simulink model "ctrlSys_mpc"  (R2025b)
settings: Solver=ode14x  StartTime=0.0  StopTime=70  FixedStep=Ts_local  RelTol=1e-4
model workspace (MAT data in the model file):
  CtrlChoice = "MPC"
values from neighbouring files (symbols this model uses):
  Ts_ctrl = 0.1    [ctrlSys.sldd]
libraries: slpidlib x1
settings Model: DataDictionary=ctrlSys.sldd  SimulationMode=accelerator  Creator=LYG  LastModifiedBy=mercer
settings SolverCC: ZeroCrossControl=DisableAll

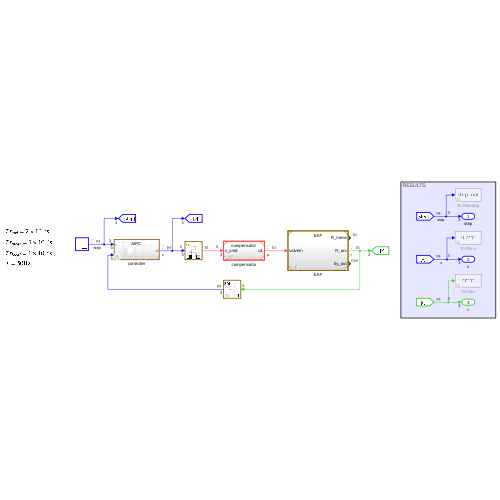
[thumbnail: Simulink's stored preview of the top-level diagram]
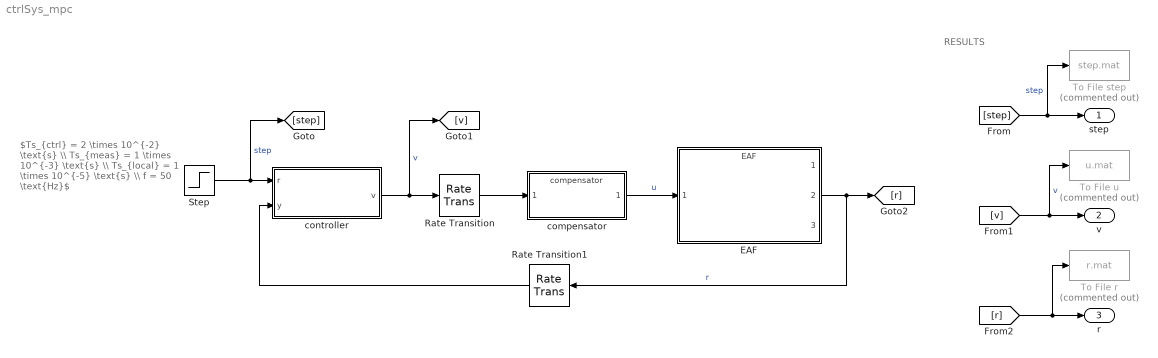
== system ctrlSys_mpc ==
  note: RESULTS
  note: $Ts_{ctrl} = 2 \times 10^{-2} \text{s} \\ Ts_{meas} = 1 \times 10^{-3} \text{s} \\ Ts_{local} = 1 \times 10^{-5} \text{s} \\ f = 50 \text{Hz}$
  EAF : ModelReference  ModelNameDialog=EAF.slx  SimulationMode=Normal  ModelReferenceVersion=1.78
  Rate Transition : RateTransition  OutPortSampleTime=Ts_local
  Rate Transition1 : RateTransition  OutPortSampleTime=Ts_ctrl
  Step : Step  Time=[35 20 50]  Before=[0.06 0.055 0.09]  After=[0.05 0.065 0.10]  SampleTime=Ts_ctrl
  To File r : ToFile  Commented=on  Filename=r.mat  MatrixName=r  SaveFormat=Timeseries
  To File step : ToFile  Commented=on  Filename=step.mat  MatrixName=step  SaveFormat=Timeseries
  To File u : ToFile  Commented=on  Filename=u.mat  MatrixName=u  SaveFormat=Timeseries
  compensator : ModelReference  ModelNameDialog=compensator.slx  SimulationMode=Normal  ModelReferenceVersion=1.22
  controller : Subsystem  Variant=on
  step : Outport
  v : Outport  Port=2
  r : Outport  Port=3
  wires:
  controller/1(v) -> [v], Rate Transition/1  "v"
  Step/1 -> controller/1(r), [step]  "step"
  Rate Transition1/1 -> controller/2(y)
  [step] -> To File step/1, step/1  "step"
  [v] -> To File u/1, v/1  "v"
  [r] -> To File r/1, r/1
  EAF/2 -> Rate Transition1/1, [r]  "r"
  Rate Transition/1 -> compensator/1
  compensator/1 -> EAF/1  "u"

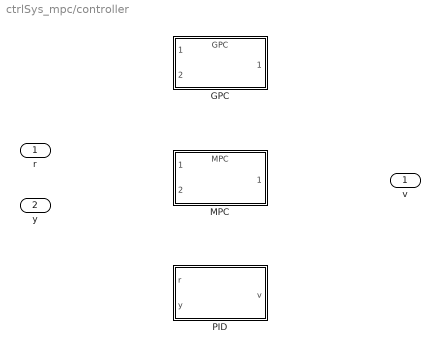
== system ctrlSys_mpc/controller ==
  r : Inport
  y : Inport  Port=2
  GPC : ModelReference  ModelNameDialog=GPC.slx  VariantControl="CtrlChoice == \"GPC\""  ModelReferenceVersion=1.211
  MPC : ModelReference  ModelNameDialog=MPC.slx  VariantControl="CtrlChoice == \"MPC\""  ModelReferenceVersion=1.7
  PID : Subsystem  VariantControl="CtrlChoice == \"PID\""
  v : Outport

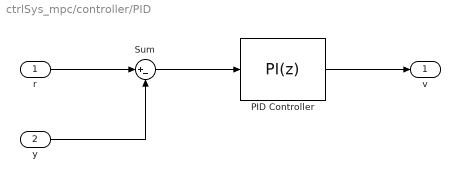
== system ctrlSys_mpc/controller/PID ==
  r : Inport
  y : Inport  Port=2
  PID Controller : slpidlib/PID Controller  Controller=PI  Form=Parallel  TimeDomain=Discrete-time  UseExternalTs=off  SampleTime=Ts_ctrl  IntegratorMethod=Forward Euler  FilterMethod=Forward Euler  ControllerParametersSource=internal  P=100  I=30  UseKiTs=off  D=0  UseExternalDerivativeSource=off  N=100  UseFilter=on  TunerSelectOption=Transfer Function Based (PID Tuner App)  InitialConditionSource=internal  InitialConditionForIntegrator=0  InitialConditionForFilter=0  DifferentiatorICPrevScaledInput=0  ExternalReset=none  TrackingMode=off  Kt=1  LimitOutput=off  SatLimitsSource=internal  UpperSaturationLimit=inf  LowerSaturationLimit=-inf  LinearizeAsGain=on  AntiWindupMode=none  Kb=1  LimitIntegrator=off  UpperIntegratorSaturationLimit=inf  LowerIntegratorSaturationLimit=-inf  POutMin=[]  POutMax=[]  IOutMin=[]  IOutMax=[]  DOutMin=[]  DOutMax=[]  NOutMin=[]  NOutMax=[]  SumOutMin=[]  SumOutMax=[]  SaturationOutMin=[]  SaturationOutMax=[]  PParamMin=[]  PParamMax=[]  IParamMin=[]  IParamMax=[]  DParamMin=[]  DParamMax=[]  NParamMin=[]  NParamMax=[]  KbParamMin=[]  KbParamMax=[]  KtParamMin=[]  KtParamMax=[]  KbOutMin=[]  KbOutMax=[]  KtOutMin=[]  KtOutMax=[]  IntegratorOutMin=[]  IntegratorOutMax=[]  FilterOutMin=[]  FilterOutMax=[]  SumI1OutMin=[]  SumI1OutMax=[]  SumI2OutMin=[]  SumI2OutMax=[]  SumI3OutMin=[]  SumI3OutMax=[]  SumI4OutMin=[]  SumI4OutMax=[]  SumDOutMin=[]  SumDOutMax=[]  DifferentiatorOutMin=[]  DifferentiatorOutMax=[]  FilterDiffOutCoefMin=[]  FilterDiffOutCoefMax=[]  ReciprocalOutMin=[]  ReciprocalOutMax=[]  SumDenOutMin=[]  SumDenOutMax=[]  SumNumOutMin=[]  SumNumOutMax=[]  DivideOutMin=[]  DivideOutMax=[]  UdiffTsProdOutMin=[]  UdiffTsProdOutMax=[]  NTsProdOutMin=[]  NTsProdOutMax=[]  UintegralTsProdOutMin=[]  UintegralTsProdOutMax=[]  UngainTsProdOutMin=[]  UngainTsProdOutMax=[]  ClampingZeroOutDataTypeStr=Inherit: Inherit via back propagation  ClampingZeroOutMin=[]  ClampingZeroOutMax=[]  FilterDenConstantOutDataTypeStr=Inherit: Inherit via back propagation  FilterDenConstantOutMin=[]  FilterDenConstantOutMax=[]  PCopyOutDataTypeStr=Inherit: Inherit via back propagation  PCopyOutMin=[]  PCopyOutMax=[]  NCopyOutDataTypeStr=Inherit: Inherit via back propagation  NCopyOutMin=[]  NCopyOutMax=[]  IntegratorContinuousStateAttributes=''  IntegratorStateMustResolveToSignalObject=off  IntegratorRTWStateStorageClass=Auto  FilterContinuousStateAttributes=''  FilterStateMustResolveToSignalObject=off  FilterRTWStateStorageClass=Auto  ParallelPVariant=InternalParameters  IdealPVariant=Disabled  IVariant=InternalParameters  DVariant=Disabled  IntegratorVariant=Discrete  SatVariant=Disabled  AWVariant=Passthrough  PCopyVariant=Disabled  TRVariant=Disabled  FdbkBlocksVariant=Forward  IdealPFdbkVariant=Disabled  SatFdbkVariant=Disabled  DerivativeFilterVariant=Disabled  NVariant=Disabled  NCopyVariant=Disabled_SignalSpec  FilterICVariant=Disabled  IntegratorICVariant=InternalICs  ExternalResetVariant=Disabled  TRSumVariant=Passthrough  SumFdbkVariant=Disabled  SumVariant=Sum_PI  TsampFilterVariant=InternalTs  TsampNgainVariant=Passthrough  TsampIntegralVariant=Disabled_SignalSpec  ExternalSaturationOutDataTypeStr=Inherit: Same as second input  DerivativeSourceVariant=Disabled  PreIntVariant=InternalPreInt
  Sum : Sum  Inputs=|+-
  v : Outport
  wires:
  r/1 -> Sum/1
  Sum/1 -> PID Controller/1
  y/1 -> Sum/2
  PID Controller/1 -> v/1
